simulink model "cartPole_Feedforward_2023b_mdl"  (R2023b)
settings: Solver=ode4  StartTime=0.0  StopTime=9  FixedStep=.001  RelTol=1e-3
undefined symbols (not defined in the file): F_x, G_f, G_theta, G_x, M, p_11, p_21
libraries: simulink_extras x1
settings Model: Creator=mo780715  LastModifiedBy=mohammadodeh
settings OptimizationCC: ReuseModelBlockBuffer=off

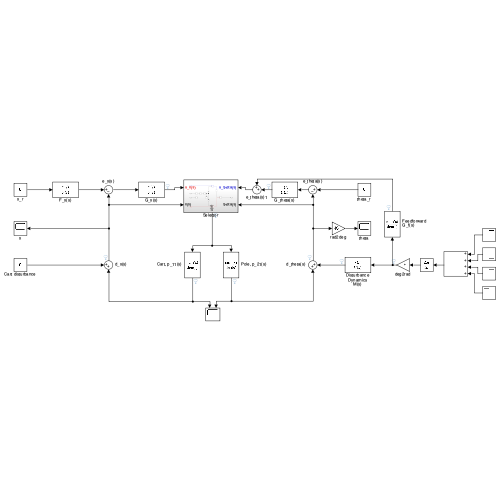
[thumbnail: Simulink's stored preview of the top-level diagram]
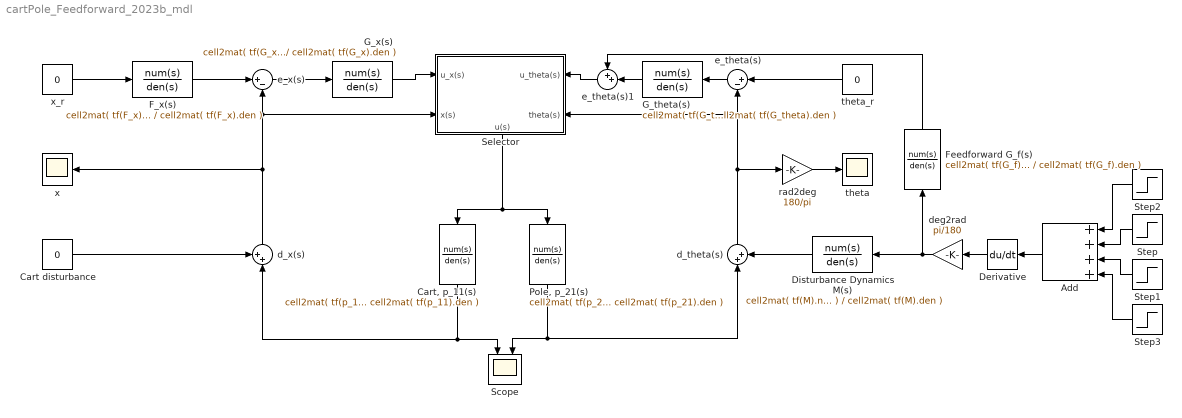
== system cartPole_Feedforward_2023b_mdl ==
  Add : Sum  Inputs=++++
  Cart disturbance : Constant  Value=0
  "Cart, p_11(s)" : TransferFcn  Numerator=cell2mat( tf(p_11).num )  Denominator=cell2mat( tf(p_11).den )  ContinuousStateAttributes='x'
  Derivative : Derivative
  Disturbance Dynamics M(s) : TransferFcn  Numerator=cell2mat( tf(M).num )  Denominator=cell2mat( tf(M).den )  ContinuousStateAttributes='theta'
  F_x(s) : TransferFcn  Numerator=cell2mat( tf(F_x).num )  Denominator=cell2mat( tf(F_x).den )
  Feedforward G_f(s) : TransferFcn  Numerator=cell2mat( tf(G_f).num )  Denominator=cell2mat( tf(G_f).den )  ContinuousStateAttributes='theta'
  G_theta(s) : TransferFcn  Numerator=cell2mat( tf(G_theta).num )  Denominator=cell2mat( tf(G_theta).den )  ContinuousStateAttributes='theta'
  G_x(s) : TransferFcn  Numerator=cell2mat( tf(G_x).num )  Denominator=cell2mat( tf(G_x).den )  ContinuousStateAttributes='x'
  "Pole, p_21(s)" : TransferFcn  Numerator=cell2mat( tf(p_21).num )  Denominator=cell2mat( tf(p_21).den )  ContinuousStateAttributes='theta'
  Scope : Scope  NumInputPorts=2
  Selector : Subsystem
      settings: PortSchema="{\"entries\":[{\"content\":{\"sides\":[{\"content\":{\"connectorIds\":[\"In1\",\"In2\"]},\"type\":\"ConnectorPlacement.EquallySpacedRectSide\",\"uuid\":\"6eba6562-edf1-4e51-babe-8905d1be8121\"},{\"content\":{\"connectorIds\":[\"In3\",\"In4\"],\"side\":\"RIGHT\"},\"type\":\"ConnectorPlacement.EquallySpacedRectSide\",\"uuid\":\"8e7a2c38-cbd1-463b-9abb-b2b1ed62e499\"},{\"content\":{\"connectorIds\":[],\"side\":\"TOP\"},\"type\":\"ConnectorPlacement.EquallySpacedRectSide\",\"uuid\":\"19fbaa4b-37e5-47c1-8c91-e7a6a78d79a5\"},{\"content\":{\"connectorIds\":[\"Out1\"],\"side\":\"BOTTOM\"},\"type\":\"ConnectorPlacement.EquallySpacedRectSide\",\"uuid\":\"f1978724-6441-4086-920a-6ea54173bdca\"}]},\"type\":\"ConnectorPlacement.EquallySpacedConnector\",\"uuid\":\"654af038-4002-438a-a48f-cf722b478931\"}],\"packageUris\":[\"http://schema.mathworks.com/mf0/Connector/R2020b\"],\"version\":\"1.0\"}"
  Step : Step  Time=3  After=-0.1  SampleTime=0
  Step1 : Step  Time=5  After=0.2  SampleTime=0
  Step2 : Step  After=0.1  SampleTime=0
  Step3 : Step  Time=7  After=-0.2  SampleTime=0
  d_theta(s) : Sum  Inputs=|++
  d_x(s) : Sum  Inputs=++|
  deg2rad : Gain  Gain=pi/180
  e_theta(s) : Sum  Inputs=|+-
  e_theta(s)1 : Sum  Inputs=++|
  e_x(s) : Sum  Inputs=|+-
  rad2deg : Gain  Gain=180/pi
  theta : Scope
  theta_r : Constant  Value=0
  x : Scope
  x_r : Constant  Value=0
  wires:
  x_r/1 -> F_x(s)/1
  "Cart, p_11(s)"/1 -> Scope/1, d_x(s)/2
  F_x(s)/1 -> e_x(s)/1
  theta_r/1 -> e_theta(s)/1
  e_x(s)/1 -> G_x(s)/1
  G_x(s)/1 -> Selector/1(u_x(s))
  d_x(s)/1 -> x/1, Selector/2(x(s)), e_x(s)/2
  Cart disturbance/1 -> d_x(s)/1
  deg2rad/1 -> Disturbance Dynamics M(s)/1, Feedforward G_f(s)/1
  e_theta(s)/1 -> G_theta(s)/1
  "Pole, p_21(s)"/1 -> Scope/2, d_theta(s)/1
  d_theta(s)/1 -> rad2deg/1, e_theta(s)/2, Selector/4(theta(s))
  rad2deg/1 -> theta/1
  Selector/1(u(s)) -> "Cart, p_11(s)"/1, "Pole, p_21(s)"/1
  Disturbance Dynamics M(s)/1 -> d_theta(s)/2
  e_theta(s)1/1 -> Selector/3(u_theta(s))
  G_theta(s)/1 -> e_theta(s)1/2
  Feedforward G_f(s)/1 -> e_theta(s)1/1
  Derivative/1 -> deg2rad/1
  Add/1 -> Derivative/1
  Step2/1 -> Add/1
  Step/1 -> Add/2
  Step1/1 -> Add/3
  Step3/1 -> Add/4

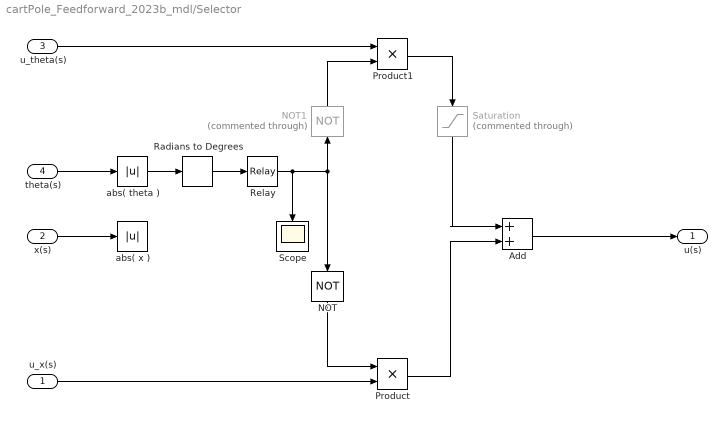
== system cartPole_Feedforward_2023b_mdl/Selector ==
  u_x(s) : Inport
  x(s) : Inport  Port=2
  u_theta(s) : Inport  Port=3
  theta(s) : Inport  Port=4
  Add : Sum
  NOT : Logic  Operator=NOT  IconShape=distinctive  AllPortsSameDT=off  OutDataTypeStr=boolean
  NOT1 : Logic  Commented=through  Operator=NOT  IconShape=distinctive  AllPortsSameDT=off  OutDataTypeStr=boolean
  Product : Product
  Product1 : Product
  Radians to Degrees : simulink_extras/Transformations/Radians to Degrees
  Relay : Relay  OnSwitchValue=0.1  OffSwitchValue=0.001
  Saturation : Saturate  Commented=through  UpperLimit=10  LowerLimit=-10
  Scope : Scope
  abs( theta ) : Abs  SaturateOnIntegerOverflow=off
  abs( x ) : Abs  SaturateOnIntegerOverflow=off
  u(s) : Outport
  wires:
  theta(s)/1 -> abs( theta )/1
  u_x(s)/1 -> Product/2
  x(s)/1 -> abs( x )/1
  abs( theta )/1 -> Radians to Degrees/1
  Radians to Degrees/1 -> Relay/1
  Add/1 -> u(s)/1
  Product/1 -> Add/2
  Relay/1 -> Scope/1, NOT1/1, NOT/1
  NOT/1 -> Product/1
  u_theta(s)/1 -> Product1/1
  Product1/1 -> Saturation/1
  NOT1/1 -> Product1/2
  Saturation/1 -> Add/1
